simulink model "OA_Dynamic"  (R2020a)
settings: Solver=VariableStepAuto  StartTime=0.0  StopTime=30  RelTol=1e-3
values from neighbouring files (symbols this model uses):
  b = 0.4    [Takeoff.m]
  body_rate_0 = [0;0;0]    [Takeoff.m]
  Boundaries = [B1;B2;B3]    [Takeoff.m]
  Euler_0 = [0;0;0]    [Takeoff.m]
  g = [0;0;-9.8]    [Takeoff.m]
  I_Drone = [0.3933,0.3933,0.76]    [Takeoff.m]
  I_Tank = CalItank(m_tank,0.4,0.1,0.4,i)    [Takeoff.m]
  J = 0.00062    [Takeoff.m]
  K = 0.074    [Takeoff.m]
  k_T = MaxMotorThrsut/(MaxRPM^2)    (= 6.99167657551e-06)    [Takeoff.m]
  k_Thrsut2Torque = 0.021    [Takeoff.m]
  l = 0.5    [Takeoff.m]
  L = sqrt((x2-x1)^2 + (y2-y1)^2)    [Takeoff.m]
  m = m_drone + m_tank*percent    (= 36)    [Takeoff.m]    (also in animation.m = T_V1toI*T_V2toV1*T_BtoV2)
  m_drone = 20    [Takeoff.m]
  m_tank = 16    [Takeoff.m]
  MaxThrust = 4*MaxMotorThrsut    (= 529.2)    [Takeoff.m]
  MaxTilt = 30*pi/180    (= 0.523598775598)    [Takeoff.m]
  MaxTorque_XY = (T2-T1)*(l/sqrt(2))    [Takeoff.m]
  MaxVolt = 48    [Takeoff.m]
  MaxYawRate = 100*pi/180    (= 1.74532925199)    [Takeoff.m]
  MaxZVel = 2    [Takeoff.m]
  percent = 1    [Takeoff.m]
  Px1 = 0.2    [Takeoff.m]
  Pz1 = 1    [Takeoff.m]
  Pz2 = 100    [Takeoff.m]
  R = 0.0062    [Takeoff.m]
  RecObstacle = [[5,4,3] ... (first row only)    [Takeoff.m]
  SafeZone = 1.0    (= 1)    [Takeoff.m]
  Target = WayPts(3,:)    [Takeoff.m]
  ts = 0.01    [Takeoff.m]
  WayPts = [[XYZ_0(1) XYZ_0(2) XYZ_0(3)] ... (first row only)    [Takeoff.m]
  XYZ_0 = [0;0;0]    [Takeoff.m]
undefined symbols (not defined in the file or in its folder): b_tank, d_drone, d_tank, DiscIntNeverNeededParam, FlyVel, h_tank, PD1, PD2, PI1, PI2, PP1, PP2, SafeFactor, Sensor0Dir, TestVel
libraries: simulink x27, vrlib x4
(part 1 of 3)
settings Model: NumberOfSteps=10  Creator=blaze8871  LastModifiedBy=blaze8871
settings DataIOCC: SaveTime=off

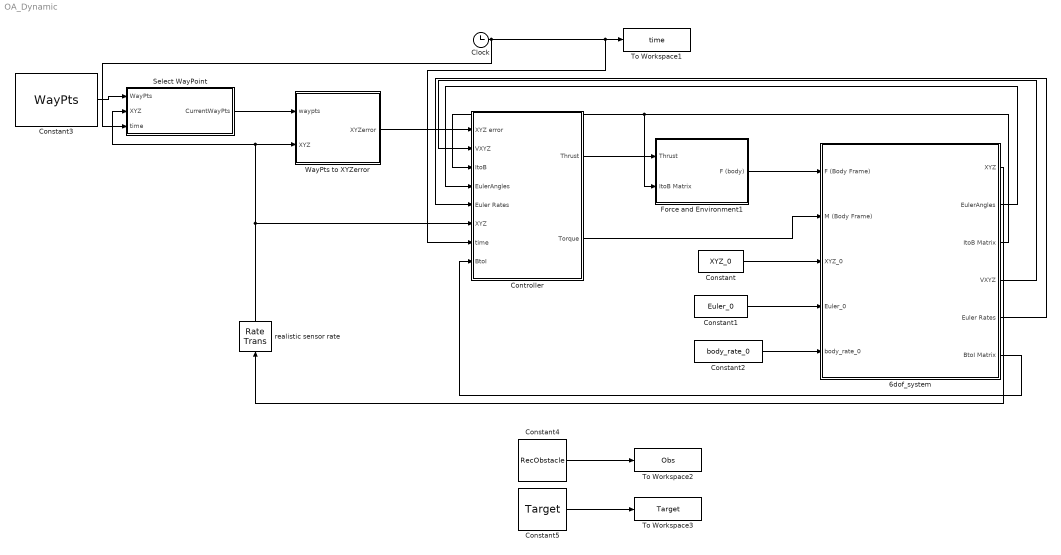
== system OA_Dynamic ==
  6dof_system : Subsystem
  Clock : Clock
  Constant : Constant  Value=XYZ_0  SampleTime=-1
  Constant1 : Constant  Value=Euler_0  SampleTime=-1
  Constant2 : Constant  Value=body_rate_0  SampleTime=-1
  Constant3 : Constant  Value=WayPts
  Constant4 : Constant  Value=RecObstacle
  Constant5 : Constant  Value=Target
  Controller : Subsystem
  Force and Environment1 : Subsystem
  Select WayPoint : Subsystem
  To Workspace1 : ToWorkspace  VariableName=time  SampleTime=ts
  To Workspace2 : ToWorkspace  VariableName=Obs  SampleTime=1000
  To Workspace3 : ToWorkspace  VariableName=Target  SampleTime=1000
  WayPts to XYZerror : MATLAB Function  TreatAsAtomicUnit=on
  realistic sensor rate : RateTransition  OutPortSampleTime=ts
  wires:
  Constant/1 -> 6dof_system/3(XYZ_0)
  Constant1/1 -> 6dof_system/4(Euler_0)
  Constant2/1 -> 6dof_system/5(body_rate_0)
  6dof_system/1(XYZ) -> realistic sensor rate/1
  6dof_system/2(EulerAngles) -> Controller/4(EulerAngles)
  WayPts to XYZerror/1(XYZerror) -> Controller/1(XYZ error)
  6dof_system/4(VXYZ) -> Controller/2(VXYZ)
  6dof_system/5(Euler Rates) -> Controller/5(Euler Rates)
  6dof_system/3(ItoB Matrix) -> Force and Environment1/2(ItoB Matrix), Controller/3(ItoB)
  Clock/1 -> Select WayPoint/3(time), Controller/7(time), To Workspace1/1
  Constant3/1 -> Select WayPoint/1(WayPts)
  realistic sensor rate/1 -> Select WayPoint/2(XYZ), WayPts to XYZerror/2(XYZ), Controller/6(XYZ)
  Select WayPoint/1(CurrentWayPts) -> WayPts to XYZerror/1(waypts)
  6dof_system/6(BtoI Matrix) -> Controller/8(BtoI)
  Controller/1(Thrust) -> Force and Environment1/1(Thrust)
  Force and Environment1/1(F (body)) -> 6dof_system/1(F (Body Frame))
  Controller/2(Torque) -> 6dof_system/2(M (Body Frame))
  Constant4/1 -> To Workspace2/1
  Constant5/1 -> To Workspace3/1

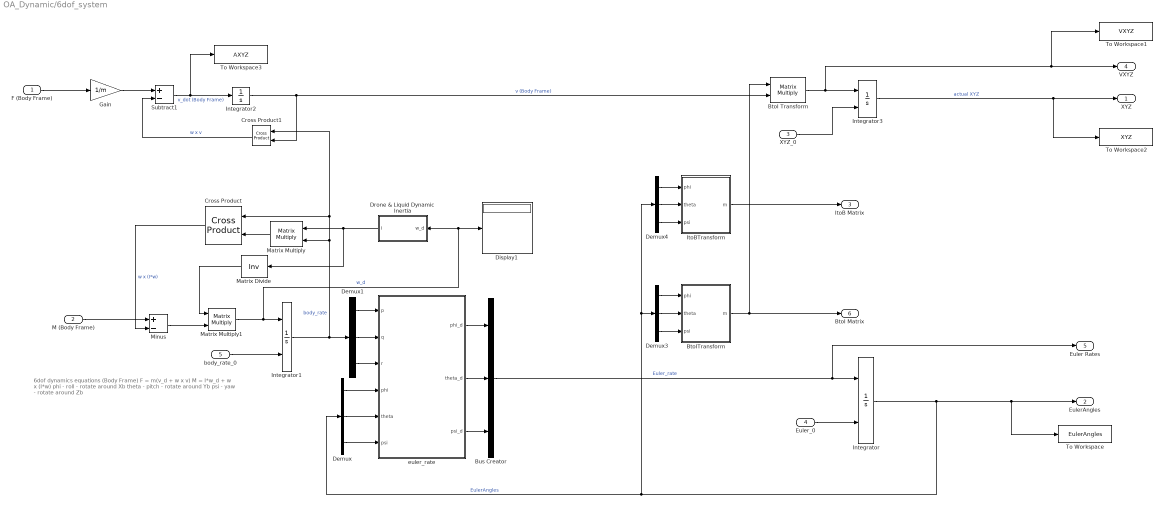
== system OA_Dynamic/6dof_system ==
  note: 6dof dynamics equations
      | (Body Frame)
      |
      | F = m(v_d + w x v)
      | M = I*w_d + w x (I*w)
      |
      | phi - roll - rotate around Xb
      | theta - pitch - rotate around Yb
      | psi - yaw - rotate around Zb
  F (Body Frame) : Inport
  M (Body Frame) : Inport  Port=2
  XYZ_0 : Inport  Port=3
  Euler_0 : Inport  Port=4
  body_rate_0 : Inport  Port=5
  BtoI Transform : Product  Multiplication=Matrix(*)
  BtoITransform : MATLAB Function  TreatAsAtomicUnit=on
  Bus Creator : BusCreator  Inputs=3
  Cross Product : vrlib/Utilities/Cross Product
  Cross Product1 : vrlib/Utilities/Cross Product
  Demux{,1,3..4} (4 alike) : Demux  Outputs=3
  Display1 : Display
  Drone & Liquid Dynamic Inertia : Subsystem
  Gain : Gain  Gain=1/m
  Integrator : Integrator  InitialConditionSource=external  ContinuousStateAttributes='EulerAngle'
  Integrator1 : Integrator  InitialConditionSource=external  ContinuousStateAttributes='EulerAngle'
  Integrator2 : Integrator
  Integrator3 : Integrator  InitialConditionSource=external
  ItoBTransform : MATLAB Function  TreatAsAtomicUnit=on
  Matrix Divide : Product  Inputs=/  Multiplication=Matrix(*)
  Matrix Multiply : Product  Multiplication=Matrix(*)
  Matrix Multiply1 : Product  Multiplication=Matrix(*)
  Minus : Sum  Inputs=+-
  Subtract1 : Sum  Inputs=+-
  To Workspace : ToWorkspace  VariableName=EulerAngles  SampleTime=ts
  To Workspace1 : ToWorkspace  VariableName=VXYZ  SampleTime=ts
  To Workspace2 : ToWorkspace  VariableName=XYZ  SampleTime=ts
  To Workspace3 : ToWorkspace  VariableName=AXYZ  SampleTime=ts
  euler_rate : MATLAB Function  TreatAsAtomicUnit=on
  XYZ : Outport
  EulerAngles : Outport  Port=2
  ItoB Matrix : Outport  Port=3
  VXYZ : Outport  Port=4
  Euler Rates : Outport  Port=5
  BtoI Matrix : Outport  Port=6
  wires:
  F (Body Frame)/1 -> Gain/1
  Demux4/2 -> ItoBTransform/2(theta)
  euler_rate/1(phi_d) -> Bus Creator/1
  BtoITransform/1(m) -> BtoI Matrix/1, BtoI Transform/1
  Bus Creator/1 -> Euler Rates/1, Integrator/1  "Euler_rate"
  Matrix Multiply/1 -> Cross Product/2
  Demux3/2 -> BtoITransform/2(theta)
  Demux/2 -> euler_rate/5(theta)
  Demux4/1 -> ItoBTransform/1(phi)
  Subtract1/1 -> To Workspace3/1, Integrator2/1  "v_dot (Body Frame)"
  Cross Product1/1 -> Subtract1/2  "w x v"
  Demux1/1 -> euler_rate/1(p)
  Demux/3 -> euler_rate/6(psi)
  euler_rate/2(theta_d) -> Bus Creator/2
  Euler_0/1 -> Integrator/2
  Integrator3/1 -> To Workspace2/1, XYZ/1  "actual XYZ"
  Cross Product/1 -> Minus/2  "w x (I*w)"
  M (Body Frame)/1 -> Minus/1
  body_rate_0/1 -> Integrator1/2
  Demux3/3 -> BtoITransform/3(psi)
  euler_rate/3(psi_d) -> Bus Creator/3
  Demux4/3 -> ItoBTransform/3(psi)
  Gain/1 -> Subtract1/1
  Demux3/1 -> BtoITransform/1(phi)
  Demux1/3 -> euler_rate/3(r)
  XYZ_0/1 -> Integrator3/2
  Demux/1 -> euler_rate/4(phi)
  Integrator2/1 -> Cross Product1/2, BtoI Transform/2  "v (Body Frame)"
  Integrator1/1 -> Cross Product1/1, Cross Product/1, Matrix Multiply/2, Demux1/1  "body_rate"
  Demux1/2 -> euler_rate/2(q)
  ItoBTransform/1(m) -> ItoB Matrix/1
  BtoI Transform/1 -> To Workspace1/1, VXYZ/1, Integrator3/1
  Minus/1 -> Matrix Multiply1/2
  Matrix Multiply1/1 -> Integrator1/1, Display1/1, Drone & Liquid Dynamic Inertia/1(w_d)  "w_d"
  Integrator/1 -> To Workspace/1, EulerAngles/1, Demux4/1, Demux3/1, Demux/1  "EulerAngles"
  Drone & Liquid Dynamic Inertia/1(I) -> Matrix Divide/1, Matrix Multiply/1
  Matrix Divide/1 -> Matrix Multiply1/1

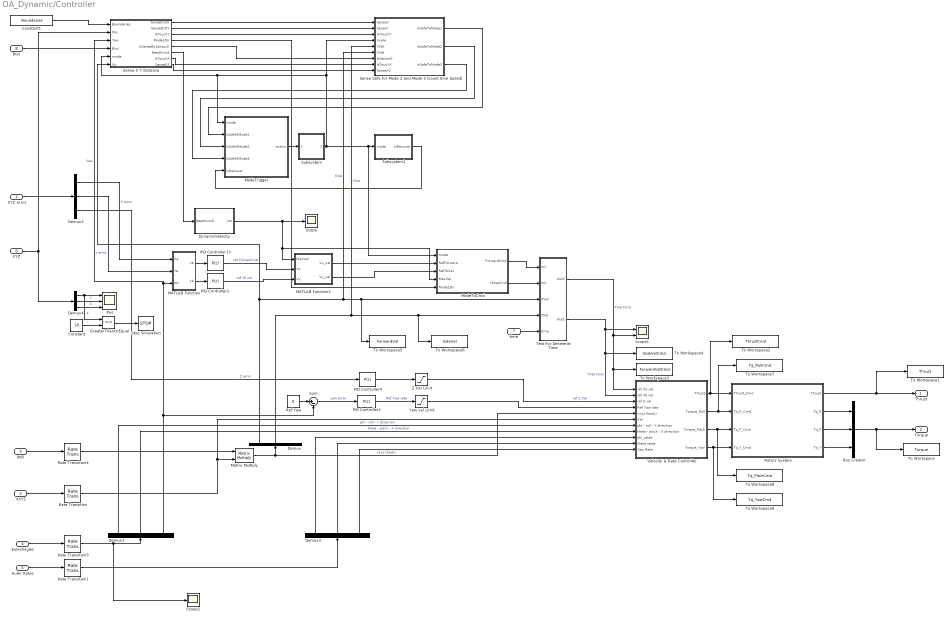
== system OA_Dynamic/Controller ==
  XYZ error : Inport
  VXYZ : Inport  Port=2
  ItoB : Inport  Port=3
  EulerAngles : Inport  Port=4
  Euler Rates : Inport  Port=5
  XYZ : Inport  Port=6
  time : Inport  Port=7
  BtoI : Inport  Port=8
  Bus Creator : BusCreator  Inputs=3
  Constant : Constant  Value=20
  Constant1 : Constant  Value=Boundaries
  Demux{,1..4} (5 alike) : Demux  Outputs=3
  DynamicVelocity : Subsystem
  GreaterThanOrEqual : RelationalOperator  OutDataTypeStr=boolean  RndMeth=Simplest
  MATLAB Function : MATLAB Function  TreatAsAtomicUnit=on
  MATLAB Function2 : MATLAB Function  TreatAsAtomicUnit=on
  Matrix Multiply : Product  Multiplication=Matrix(*)
  ModeToCmd : MATLAB Function  TreatAsAtomicUnit=on
  ModeTrigger : MATLAB Function  TreatAsAtomicUnit=on
  PID Controller1 : simulink/Continuous/PID Controller  Controller=P  Form=Parallel  TimeDomain=Discrete-time  UseExternalTs=off  SampleTime=ts  IntegratorMethod=Forward Euler  FilterMethod=Forward Euler  ControllerParametersSource=internal  P=1  I=1  D=0  UseFilter=on  N=100  TunerSelectOption=Transfer Function Based (PID Tuner App)  InitialConditionSource=internal  InitialConditionForIntegrator=0  InitialConditionForFilter=0  DifferentiatorICPrevScaledInput=0  ExternalReset=none  TrackingMode=off  Kt=1  LimitOutput=off  UpperSaturationLimit=inf  LowerSaturationLimit=-inf  LinearizeAsGain=on  AntiWindupMode=none  Kb=1  POutMin=[]  POutMax=[]  IOutMin=[]  IOutMax=[]  DOutMin=[]  DOutMax=[]  NOutMin=[]  NOutMax=[]  SumOutMin=[]  SumOutMax=[]  SaturationOutMin=[]  SaturationOutMax=[]  PParamMin=[]  PParamMax=[]  IParamMin=[]  IParamMax=[]  DParamMin=[]  DParamMax=[]  NParamMin=[]  NParamMax=[]  KbParamMin=[]  KbParamMax=[]  KtParamMin=[]  KtParamMax=[]  KbOutMin=[]  KbOutMax=[]  KtOutMin=[]  KtOutMax=[]  IntegratorOutMin=[]  IntegratorOutMax=[]  FilterOutMin=[]  FilterOutMax=[]  SumI1OutMin=[]  SumI1OutMax=[]  SumI2OutMin=[]  SumI2OutMax=[]  SumI3OutMin=[]  SumI3OutMax=[]  SumI4OutMin=[]  SumI4OutMax=[]  SumDOutMin=[]  SumDOutMax=[]  DifferentiatorOutMin=[]  DifferentiatorOutMax=[]  FilterDiffOutCoefMin=[]  FilterDiffOutCoefMax=[]  ReciprocalOutMin=[]  ReciprocalOutMax=[]  SumDenOutMin=[]  SumDenOutMax=[]  SumNumOutMin=[]  SumNumOutMax=[]  DivideOutMin=[]  DivideOutMax=[]  UdiffTsProdOutMin=[]  UdiffTsProdOutMax=[]  NTsProdOutMin=[]  NTsProdOutMax=[]  UintegralTsProdOutMin=[]  UintegralTsProdOutMax=[]  UngainTsProdOutMin=[]  UngainTsProdOutMax=[]  IntegratorContinuousStateAttributes=''  IntegratorStateMustResolveToSignalObject=off  IntegratorRTWStateStorageClass=Auto  FilterContinuousStateAttributes=''  FilterStateMustResolveToSignalObject=off  FilterRTWStateStorageClass=Auto  ParallelPVariant=InternalParameters  IdealPVariant=Disabled  IVariant=Disabled  DVariant=Disabled  IntegratorVariant=Disabled  SatVariant=Disabled  AWVariant=Disabled  PCopyVariant=Disabled  TRVariant=Disabled  FdbkBlocksVariant=Forward  IdealPFdbkVariant=Disabled  SatFdbkVariant=Disabled  DerivativeFilterVariant=Disabled  NVariant=Disabled  NCopyVariant=Disabled_SignalSpec  FilterICVariant=Disabled  IntegratorICVariant=Disabled  ExternalResetVariant=Disabled  TRSumVariant=Passthrough  SumFdbkVariant=Disabled  SumVariant=Passthrough_P  TsampFilterVariant=InternalTs  TsampNgainVariant=Passthrough  TsampIntegralVariant=Disabled_SignalSpec
  PID Controller13 : simulink/Continuous/PID Controller  Controller=P  Form=Parallel  TimeDomain=Discrete-time  UseExternalTs=off  SampleTime=ts  IntegratorMethod=Forward Euler  FilterMethod=Forward Euler  ControllerParametersSource=internal  P=0.6  I=1  D=0  UseFilter=on  N=100  TunerSelectOption=Transfer Function Based (PID Tuner App)  InitialConditionSource=internal  InitialConditionForIntegrator=0  InitialConditionForFilter=0  DifferentiatorICPrevScaledInput=0  ExternalReset=none  TrackingMode=off  Kt=1  LimitOutput=off  UpperSaturationLimit=inf  LowerSaturationLimit=-inf  LinearizeAsGain=on  AntiWindupMode=none  Kb=1  POutMin=[]  POutMax=[]  IOutMin=[]  IOutMax=[]  DOutMin=[]  DOutMax=[]  NOutMin=[]  NOutMax=[]  SumOutMin=[]  SumOutMax=[]  SaturationOutMin=[]  SaturationOutMax=[]  PParamMin=[]  PParamMax=[]  IParamMin=[]  IParamMax=[]  DParamMin=[]  DParamMax=[]  NParamMin=[]  NParamMax=[]  KbParamMin=[]  KbParamMax=[]  KtParamMin=[]  KtParamMax=[]  KbOutMin=[]  KbOutMax=[]  KtOutMin=[]  KtOutMax=[]  IntegratorOutMin=[]  IntegratorOutMax=[]  FilterOutMin=[]  FilterOutMax=[]  SumI1OutMin=[]  SumI1OutMax=[]  SumI2OutMin=[]  SumI2OutMax=[]  SumI3OutMin=[]  SumI3OutMax=[]  SumI4OutMin=[]  SumI4OutMax=[]  SumDOutMin=[]  SumDOutMax=[]  DifferentiatorOutMin=[]  DifferentiatorOutMax=[]  FilterDiffOutCoefMin=[]  FilterDiffOutCoefMax=[]  ReciprocalOutMin=[]  ReciprocalOutMax=[]  SumDenOutMin=[]  SumDenOutMax=[]  SumNumOutMin=[]  SumNumOutMax=[]  DivideOutMin=[]  DivideOutMax=[]  UdiffTsProdOutMin=[]  UdiffTsProdOutMax=[]  NTsProdOutMin=[]  NTsProdOutMax=[]  UintegralTsProdOutMin=[]  UintegralTsProdOutMax=[]  UngainTsProdOutMin=[]  UngainTsProdOutMax=[]  IntegratorContinuousStateAttributes=''  IntegratorStateMustResolveToSignalObject=off  IntegratorRTWStateStorageClass=Auto  FilterContinuousStateAttributes=''  FilterStateMustResolveToSignalObject=off  FilterRTWStateStorageClass=Auto  ParallelPVariant=InternalParameters  IdealPVariant=Disabled  IVariant=Disabled  DVariant=Disabled  IntegratorVariant=Disabled  SatVariant=Disabled  AWVariant=Disabled  PCopyVariant=Disabled  TRVariant=Disabled  FdbkBlocksVariant=Forward  IdealPFdbkVariant=Disabled  SatFdbkVariant=Disabled  DerivativeFilterVariant=Disabled  NVariant=Disabled  NCopyVariant=Disabled_SignalSpec  FilterICVariant=Disabled  IntegratorICVariant=Disabled  ExternalResetVariant=Disabled  TRSumVariant=Passthrough  SumFdbkVariant=Disabled  SumVariant=Passthrough_P  TsampFilterVariant=InternalTs  TsampNgainVariant=Passthrough  TsampIntegralVariant=Disabled_SignalSpec
  PID Controller2 : simulink/Continuous/PID Controller  Controller=P  Form=Parallel  TimeDomain=Discrete-time  UseExternalTs=off  SampleTime=ts  IntegratorMethod=Forward Euler  FilterMethod=Forward Euler  ControllerParametersSource=internal  P=0.6  I=1  D=0  UseFilter=on  N=100  TunerSelectOption=Transfer Function Based (PID Tuner App)  InitialConditionSource=internal  InitialConditionForIntegrator=0  InitialConditionForFilter=0  DifferentiatorICPrevScaledInput=0  ExternalReset=none  TrackingMode=off  Kt=1  LimitOutput=off  UpperSaturationLimit=inf  LowerSaturationLimit=-inf  LinearizeAsGain=on  AntiWindupMode=none  Kb=1  POutMin=[]  POutMax=[]  IOutMin=[]  IOutMax=[]  DOutMin=[]  DOutMax=[]  NOutMin=[]  NOutMax=[]  SumOutMin=[]  SumOutMax=[]  SaturationOutMin=[]  SaturationOutMax=[]  PParamMin=[]  PParamMax=[]  IParamMin=[]  IParamMax=[]  DParamMin=[]  DParamMax=[]  NParamMin=[]  NParamMax=[]  KbParamMin=[]  KbParamMax=[]  KtParamMin=[]  KtParamMax=[]  KbOutMin=[]  KbOutMax=[]  KtOutMin=[]  KtOutMax=[]  IntegratorOutMin=[]  IntegratorOutMax=[]  FilterOutMin=[]  FilterOutMax=[]  SumI1OutMin=[]  SumI1OutMax=[]  SumI2OutMin=[]  SumI2OutMax=[]  SumI3OutMin=[]  SumI3OutMax=[]  SumI4OutMin=[]  SumI4OutMax=[]  SumDOutMin=[]  SumDOutMax=[]  DifferentiatorOutMin=[]  DifferentiatorOutMax=[]  FilterDiffOutCoefMin=[]  FilterDiffOutCoefMax=[]  ReciprocalOutMin=[]  ReciprocalOutMax=[]  SumDenOutMin=[]  SumDenOutMax=[]  SumNumOutMin=[]  SumNumOutMax=[]  DivideOutMin=[]  DivideOutMax=[]  UdiffTsProdOutMin=[]  UdiffTsProdOutMax=[]  NTsProdOutMin=[]  NTsProdOutMax=[]  UintegralTsProdOutMin=[]  UintegralTsProdOutMax=[]  UngainTsProdOutMin=[]  UngainTsProdOutMax=[]  IntegratorContinuousStateAttributes=''  IntegratorStateMustResolveToSignalObject=off  IntegratorRTWStateStorageClass=Auto  FilterContinuousStateAttributes=''  FilterStateMustResolveToSignalObject=off  FilterRTWStateStorageClass=Auto  ParallelPVariant=InternalParameters  IdealPVariant=Disabled  IVariant=Disabled  DVariant=Disabled  IntegratorVariant=Disabled  SatVariant=Disabled  AWVariant=Disabled  PCopyVariant=Disabled  TRVariant=Disabled  FdbkBlocksVariant=Forward  IdealPFdbkVariant=Disabled  SatFdbkVariant=Disabled  DerivativeFilterVariant=Disabled  NVariant=Disabled  NCopyVariant=Disabled_SignalSpec  FilterICVariant=Disabled  IntegratorICVariant=Disabled  ExternalResetVariant=Disabled  TRSumVariant=Passthrough  SumFdbkVariant=Disabled  SumVariant=Passthrough_P  TsampFilterVariant=InternalTs  TsampNgainVariant=Passthrough  TsampIntegralVariant=Disabled_SignalSpec
  PID Controller4 : simulink/Continuous/PID Controller  Controller=P  Form=Parallel  TimeDomain=Discrete-time  UseExternalTs=off  SampleTime=ts  IntegratorMethod=Forward Euler  FilterMethod=Forward Euler  ControllerParametersSource=internal  P=Pz1  I=1  D=0  UseFilter=on  N=100  TunerSelectOption=Transfer Function Based (PID Tuner App)  InitialConditionSource=internal  InitialConditionForIntegrator=0  InitialConditionForFilter=0  DifferentiatorICPrevScaledInput=0  ExternalReset=none  TrackingMode=off  Kt=1  LimitOutput=off  UpperSaturationLimit=inf  LowerSaturationLimit=-inf  LinearizeAsGain=on  AntiWindupMode=none  Kb=1  POutMin=[]  POutMax=[]  IOutMin=[]  IOutMax=[]  DOutMin=[]  DOutMax=[]  NOutMin=[]  NOutMax=[]  SumOutMin=[]  SumOutMax=[]  SaturationOutMin=[]  SaturationOutMax=[]  PParamMin=[]  PParamMax=[]  IParamMin=[]  IParamMax=[]  DParamMin=[]  DParamMax=[]  NParamMin=[]  NParamMax=[]  KbParamMin=[]  KbParamMax=[]  KtParamMin=[]  KtParamMax=[]  KbOutMin=[]  KbOutMax=[]  KtOutMin=[]  KtOutMax=[]  IntegratorOutMin=[]  IntegratorOutMax=[]  FilterOutMin=[]  FilterOutMax=[]  SumI1OutMin=[]  SumI1OutMax=[]  SumI2OutMin=[]  SumI2OutMax=[]  SumI3OutMin=[]  SumI3OutMax=[]  SumI4OutMin=[]  SumI4OutMax=[]  SumDOutMin=[]  SumDOutMax=[]  DifferentiatorOutMin=[]  DifferentiatorOutMax=[]  FilterDiffOutCoefMin=[]  FilterDiffOutCoefMax=[]  ReciprocalOutMin=[]  ReciprocalOutMax=[]  SumDenOutMin=[]  SumDenOutMax=[]  SumNumOutMin=[]  SumNumOutMax=[]  DivideOutMin=[]  DivideOutMax=[]  UdiffTsProdOutMin=[]  UdiffTsProdOutMax=[]  NTsProdOutMin=[]  NTsProdOutMax=[]  UintegralTsProdOutMin=[]  UintegralTsProdOutMax=[]  UngainTsProdOutMin=[]  UngainTsProdOutMax=[]  IntegratorContinuousStateAttributes=''  IntegratorStateMustResolveToSignalObject=off  IntegratorRTWStateStorageClass=Auto  FilterContinuousStateAttributes=''  FilterStateMustResolveToSignalObject=off  FilterRTWStateStorageClass=Auto  ParallelPVariant=InternalParameters  IdealPVariant=Disabled  IVariant=Disabled  DVariant=Disabled  IntegratorVariant=Disabled  SatVariant=Disabled  AWVariant=Disabled  PCopyVariant=Disabled  TRVariant=Disabled  FdbkBlocksVariant=Forward  IdealPFdbkVariant=Disabled  SatFdbkVariant=Disabled  DerivativeFilterVariant=Disabled  NVariant=Disabled  NCopyVariant=Disabled_SignalSpec  FilterICVariant=Disabled  IntegratorICVariant=Disabled  ExternalResetVariant=Disabled  TRSumVariant=Passthrough  SumFdbkVariant=Disabled  SumVariant=Passthrough_P  TsampFilterVariant=InternalTs  TsampNgainVariant=Passthrough  TsampIntegralVariant=Disabled_SignalSpec
  Pos : Scope  NumInputPorts=3
  Rate Transition{,1,3..4} (4 alike) : RateTransition  OutPortSampleTime=ts
  Ref Yaw : Constant  Value=0
  Rotors System : Subsystem
  Scope : Scope
  Scope1 : Scope  NumInputPorts=2
  Scope2 : Scope
  Sense Safe for Mode 2 and Mode 3 (count time based) : Subsystem
  Sense X Y Distance : Subsystem
  Stop Simulation : Stop
  Subsystem : Subsystem
  Subsystem1 : Subsystem
  Sum : Sum  Inputs=|+-
  Test For Decelerat Time : Subsystem
  To Workspace : ToWorkspace  VariableName=Torque  SampleTime=ts
  To Workspace1 : ToWorkspace  VariableName=Thrust  SampleTime=ts
  To Workspace2 : ToWorkspace  VariableName=ThrustCmd  SampleTime=ts
  To Workspace3 : ToWorkspace  VariableName=ForwardVelCmd  SampleTime=ts
  To Workspace4 : ToWorkspace  VariableName=SideVelCmd  SampleTime=ts
  To Workspace5 : ToWorkspace  VariableName=ForwardVel  SampleTime=ts
  To Workspace6 : ToWorkspace  VariableName=SideVel  SampleTime=ts
  To Workspace7 : ToWorkspace  VariableName=Tq_RollCmd  SampleTime=ts
  To Workspace8 : ToWorkspace  VariableName=Tq_PitchCmd  SampleTime=ts
  To Workspace9 : ToWorkspace  VariableName=Tq_YawCmd  SampleTime=ts
  Velocity & Rate Controller : Subsystem
  Yaw vel Limit : Saturate  UpperLimit=MaxYawRate  LowerLimit=-MaxYawRate
  Z Vel Limit : Saturate  UpperLimit=MaxZVel  LowerLimit=-MaxZVel
  Thrust : Outport
  Torque : Outport  Port=2
  wires:
  Bus Creator/1 -> To Workspace/1, Torque/1
  VXYZ/1 -> Rate Transition/1
  Demux2/3 -> PID Controller4/1  "Z error"
  EulerAngles/1 -> Rate Transition3/1
  Demux1/3 -> MATLAB Function/3(psi), Sense X Y Distance/3(Yaw), Sum/2  "Yaw"
  Sum/1 -> PID Controller1/1  "yaw error"
  ItoB/1 -> Rate Transition4/1
  XYZ error/1 -> Demux2/1
  Rate Transition3/1 -> Scope2/1, Demux1/1
  Rate Transition4/1 -> Matrix Multiply/1
  Euler Rates/1 -> Rate Transition1/1
  Rate Transition1/1 -> Demux3/1
  Demux2/1 -> MATLAB Function/1(Xe)  "X error"
  Demux2/2 -> MATLAB Function/2(Ye)  "y error"
  Rate Transition/1 -> Velocity & Rate Controller/6(Vel), Matrix Multiply/2
  MATLAB Function/1(xb) -> PID Controller13/1
  PID Controller13/1 -> MATLAB Function2/2(Vx)  "ref Forward vel"
  Matrix Multiply/1 -> Velocity & Rate Controller/5(vxyz (body)), Demux/1  "vxyz (body)"
  PID Controller4/1 -> Z Vel Limit/1
  PID Controller1/1 -> Yaw vel Limit/1  "Ref Yaw rate"
  Demux1/1 -> Velocity & Rate Controller/7(phi - roll - Y direction)  "phi - roll - Y direction"
  Demux1/2 -> Velocity & Rate Controller/8(theta - pitch - X direction)  "theta - pitch - X direction"
  Demux3/1 -> Velocity & Rate Controller/9(phi_rates)
  Demux3/2 -> Velocity & Rate Controller/10(theta rates)
  Demux3/3 -> Velocity & Rate Controller/11(Yaw Rate)
  MATLAB Function2/1(Vx_cal) -> ModeToCmd/2(RefForward)
  Yaw vel Limit/1 -> Velocity & Rate Controller/4(Ref Yaw rate)
  Ref Yaw/1 -> Sum/1
  MATLAB Function/2(yb) -> PID Controller2/1
  PID Controller2/1 -> MATLAB Function2/3(Vy)  "ref Yb vel"
  MATLAB Function2/2(Vy_cal) -> ModeToCmd/3(RefYbVel)
  XYZ/1 -> Sense X Y Distance/2(Pos), Demux4/1
  Demux4/1 -> GreaterThanOrEqual/1, Pos/1  "X"
  Demux4/2 -> Pos/2  "Y"
  Demux4/3 -> Pos/3  "Z"
  Demux/2 -> Sense Safe for Mode 2 and Mode 3 (count time based)/5(YVel), To Workspace6/1, Test For Decelerat Time/4(YVel)  "YVel"
  Demux/1 -> Sense X Y Distance/6(Vx), Sense Safe for Mode 2 and Mode 3 (count time based)/6(XVel), To Workspace5/1, Test For Decelerat Time/3(XVel)  "XVel"
  Sense X Y Distance/1(SenseDistX) -> Sense Safe for Mode 2 and Mode 3 (count time based)/1(SenseX)
  Constant1/1 -> Sense X Y Distance/1(Boundaries)
  Sense X Y Distance/2(SenseDistY) -> Sense Safe for Mode 2 and Mode 3 (count time based)/2(SenseY)
  Velocity & Rate Controller/1(Thrust) -> Rotors System/1(Thrust_Cmd), To Workspace2/1
  Velocity & Rate Controller/2(Torque_Roll) -> To Workspace7/1, Rotors System/2(Tq_R_Cmd)
  Velocity & Rate Controller/3(Torque_Pitch) -> To Workspace8/1, Rotors System/3(Tq_P_Cmd)
  Velocity & Rate Controller/4(Torque_Yaw) -> To Workspace9/1, Rotors System/4(Tq_Y_Cmd)
  Rotors System/1(Thrust) -> Thrust/1, To Workspace1/1
  Rotors System/2(Tq_R) -> Bus Creator/1
  Rotors System/3(Tq_P) -> Bus Creator/2
  Rotors System/4(Tq_Y) -> Bus Creator/3
  Subsystem/1(mode) -> Subsystem1/1(mode), ModeToCmd/1(mode), ModeTrigger/1(mode), Sense X Y Distance/5(mode), Sense Safe for Mode 2 and Mode 3 (count time based)/4(mode)
  ModeTrigger/1(action) -> Subsystem/1(action)
  Subsystem1/1(IsRecover) -> ModeTrigger/5(IsRecover)
  Z Vel Limit/1 -> Velocity & Rate Controller/3(ref Z vel)  "ref Z Vel"
  Sense Safe for Mode 2 and Mode 3 (count time based)/2(IsSafeToMode2) -> ModeTrigger/3(IsSafe2Mode2)
  Sense X Y Distance/3(IsTouchY) -> Sense Safe for Mode 2 and Mode 3 (count time based)/3(IsTouchY)
  Sense Safe for Mode 2 and Mode 3 (count time based)/3(IsSafeToMode3) -> ModeTrigger/4(IsSafe2Mode3)
  Test For Decelerat Time/2(Out1) -> Scope1/1, To Workspace4/1, Velocity & Rate Controller/2(ref Yb vel)  "YVel Cmd"
  Test For Decelerat Time/1(Out2) -> Scope1/2, To Workspace3/1, Velocity & Rate Controller/1(ref Xb vel)  "XVel Cmd"
  ModeToCmd/1(ForwardCmd) -> Test For Decelerat Time/1(In1)
  ModeToCmd/2(YbVelCmd) -> Test For Decelerat Time/2(In2)
  time/1 -> Test For Decelerat Time/5(time)
  Sense Safe for Mode 2 and Mode 3 (count time based)/1(IsSafeToMode1) -> ModeTrigger/2(IsSafe2Mode1)
  BtoI/1 -> Sense X Y Distance/4(BtoI)
  Sense X Y Distance/4(Mode1Dir) -> ModeToCmd/5(Mode1Dir)
  Sense X Y Distance/5(IsSenseBySensor0) -> Sense Safe for Mode 2 and Mode 3 (count time based)/7(IsSensor0)
  DynamicVelocity/1(Vel) -> Scope/1, ModeToCmd/4(MaxVel), MATLAB Function2/1(MaxVel)
  Sense X Y Distance/6(NeedAvoid) -> DynamicVelocity/1(NeedAvoid)
  Sense X Y Distance/7(IsTouchX) -> Sense Safe for Mode 2 and Mode 3 (count time based)/8(IsTouchX)
  Sense X Y Distance/8(SenseX2) -> Sense Safe for Mode 2 and Mode 3 (count time based)/9(SenseX2)
  GreaterThanOrEqual/1 -> Stop Simulation/1
  Constant/1 -> GreaterThanOrEqual/2

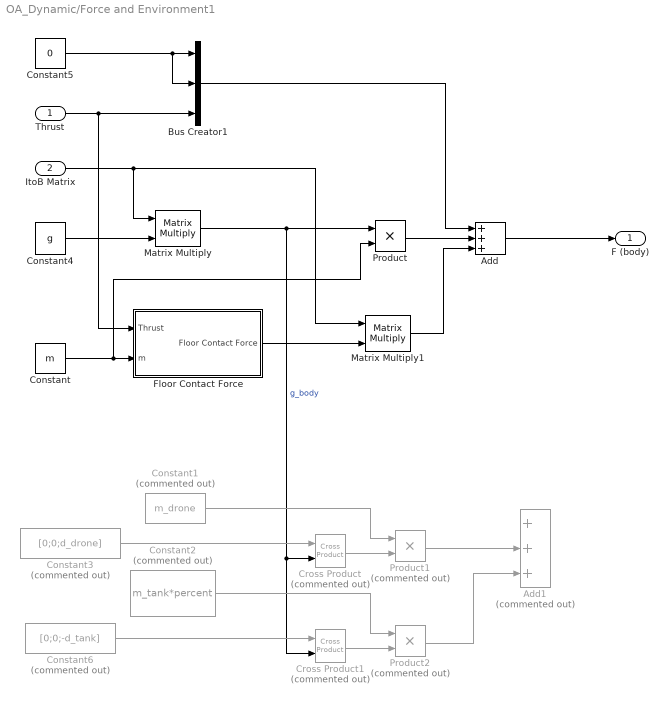
== system OA_Dynamic/Force and Environment1 ==
  Thrust : Inport
  ItoB Matrix : Inport  Port=2
  Add : Sum  Inputs=+++
  Add1 : Sum  Commented=on  Inputs=+++
  Bus Creator1 : BusCreator  Inputs=3
  Constant : Constant  Value=m  SampleTime=ts
  Constant1 : Constant  Commented=on  Value=m_drone  SampleTime=ts
  Constant2 : Constant  Commented=on  Value=m_tank*percent  SampleTime=ts
  Constant3 : Constant  Commented=on  Value=[0;0;d_drone]  SampleTime=ts
  Constant4 : Constant  Value=g  SampleTime=-1
  Constant5 : Constant  Value=0  SampleTime=-1
  Constant6 : Constant  Commented=on  Value=[0;0;-d_tank]  SampleTime=ts
  Cross Product : vrlib/Utilities/Cross Product  Commented=on
  Cross Product1 : vrlib/Utilities/Cross Product  Commented=on
  Floor Contact Force : Subsystem
  Matrix Multiply : Product  Multiplication=Matrix(*)
  Matrix Multiply1 : Product  Multiplication=Matrix(*)
  Product : Product
  Product1 : Product  Commented=on
  Product2 : Product  Commented=on
  F (body) : Outport
  wires:
  Thrust/1 -> Floor Contact Force/1(Thrust), Bus Creator1/3
  ItoB Matrix/1 -> Matrix Multiply/1, Matrix Multiply1/1
  Constant5/1 -> Bus Creator1/2, Bus Creator1/1
  Add/1 -> F (body)/1
  Constant/1 -> Product/2, Floor Contact Force/2(m)
  Bus Creator1/1 -> Add/1
  Floor Contact Force/1(Floor Contact Force) -> Matrix Multiply1/2
  Matrix Multiply1/1 -> Add/3
  Constant4/1 -> Matrix Multiply/2
  Matrix Multiply/1 -> Cross Product/2, Cross Product1/2, Product/1  "g_body"
  Product/1 -> Add/2
  Constant3/1 -> Cross Product/1
  Cross Product/1 -> Product1/2
  Constant1/1 -> Product1/1
  Cross Product1/1 -> Product2/2
  Constant6/1 -> Cross Product1/1
  Constant2/1 -> Product2/1
  Product1/1 -> Add1/2
  Product2/1 -> Add1/3

== system OA_Dynamic/Select WayPoint ==
  WayPts : Inport
  XYZ : Inport  Port=2
  time : Inport  Port=3
  Discrete-Time Integrator : DiscreteIntegrator  SampleTime=ts  ICPrevOutput=DiscIntNeverNeededParam  ICPrevScaledInput=DiscIntNeverNeededParam
  Gain : Gain  Gain=100
  MATLAB Function : MATLAB Function  TreatAsAtomicUnit=on
  MATLAB Function1 : MATLAB Function  TreatAsAtomicUnit=on
  Scope : Scope
  CurrentWayPts : Outport
  wires:
  WayPts/1 -> MATLAB Function/1(WayPts)
  MATLAB Function/1(CurrentWayPts) -> CurrentWayPts/1, MATLAB Function1/1(CurrentWayPts)
  Gain/1 -> MATLAB Function1/3(Index), MATLAB Function/2(WayPtsIndex), Scope/1
  XYZ/1 -> MATLAB Function1/2(XYZ)
  MATLAB Function1/1(TouchWayPts) -> Discrete-Time Integrator/1
  Discrete-Time Integrator/1 -> Gain/1
  time/1 -> MATLAB Function1/4(time)

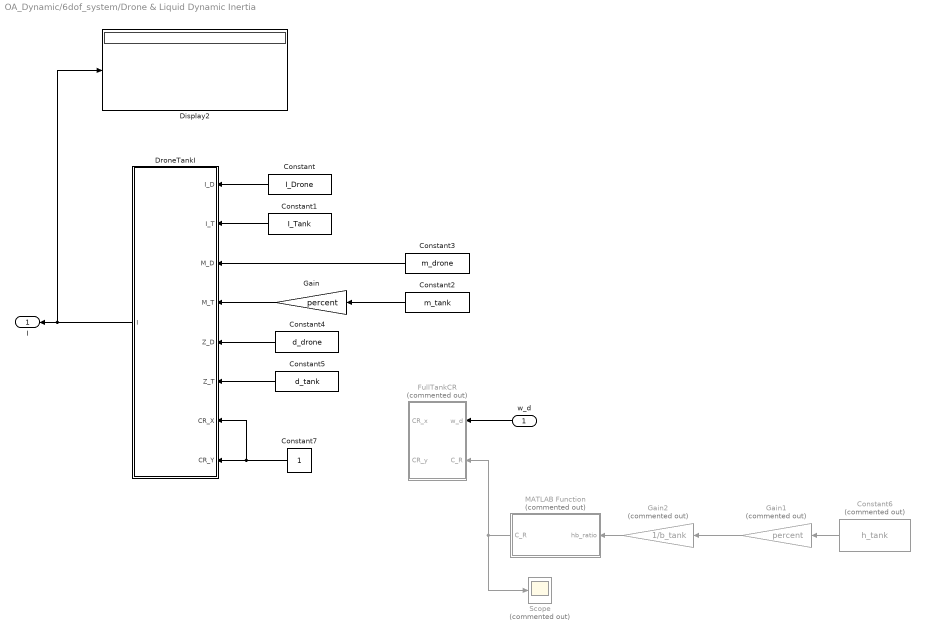
== system OA_Dynamic/6dof_system/Drone & Liquid Dynamic Inertia ==
  w_d : Inport
  Constant : Constant  Value=I_Drone
  Constant1 : Constant  Value=I_Tank
  Constant2 : Constant  Value=m_tank
  Constant3 : Constant  Value=m_drone
  Constant4 : Constant  Value=d_drone
  Constant5 : Constant  Value=d_tank
  Constant6 : Constant  Commented=on  Value=h_tank
  Constant7 : Constant
  Display2 : Display
  DroneTankI : MATLAB Function  TreatAsAtomicUnit=on
  FullTankCR : MATLAB Function  Commented=on  TreatAsAtomicUnit=on
  Gain : Gain  Gain=percent
  Gain1 : Gain  Commented=on  Gain=percent
  Gain2 : Gain  Commented=on  Gain=1/b_tank
  MATLAB Function : MATLAB Function  Commented=on  TreatAsAtomicUnit=on
  Scope : Scope  Commented=on
  I : Outport
  wires:
  Constant/1 -> DroneTankI/1(I_D)
  w_d/1 -> FullTankCR/1(w_d)
  DroneTankI/1(I) -> Display2/1, I/1
  Constant1/1 -> DroneTankI/2(I_T)
  Constant3/1 -> DroneTankI/3(M_D)
  Gain/1 -> DroneTankI/4(M_T)
  Constant2/1 -> Gain/1
  Constant4/1 -> DroneTankI/5(Z_D)
  Constant5/1 -> DroneTankI/6(Z_T)
  Constant6/1 -> Gain1/1
  Gain1/1 -> Gain2/1
  Gain2/1 -> MATLAB Function/1(hb_ratio)
  MATLAB Function/1(C_R) -> Scope/1, FullTankCR/2(C_R)
  Constant7/1 -> DroneTankI/8(CR_Y), DroneTankI/7(CR_X)

== system OA_Dynamic/Controller/DynamicVelocity ==
  NeedAvoid : Inport
  Constant : Constant  Value=percent
  Constant2 : Constant  Value=FlyVel
  MATLAB Function1 : MATLAB Function  TreatAsAtomicUnit=on
  MATLAB Function3 : MATLAB Function  TreatAsAtomicUnit=on
  To Workspace2 : ToWorkspace  VariableName=P_LQ  SampleTime=1000
  Vel : Outport
  wires:
  MATLAB Function3/1(Vel) -> Vel/1
  NeedAvoid/1 -> MATLAB Function3/1(NeedAvoid)
  Constant2/1 -> MATLAB Function3/2(FlyVel)
  MATLAB Function1/1(MaxVel) -> MATLAB Function3/3(MaxVel)
  Constant/1 -> To Workspace2/1, MATLAB Function1/1(WaterLevel)

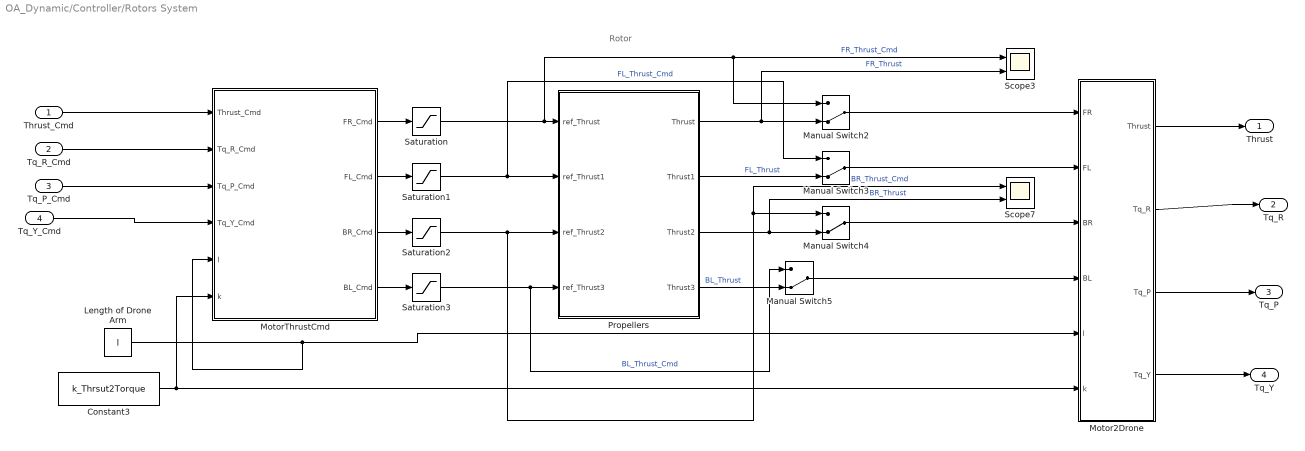
== system OA_Dynamic/Controller/Rotors System ==
  note: Rotor
  Thrust_Cmd : Inport
  Tq_R_Cmd : Inport  Port=2
  Tq_P_Cmd : Inport  Port=3
  Tq_Y_Cmd : Inport  Port=4
  Constant3 : Constant  Value=k_Thrsut2Torque
  Length of Drone Arm : Constant  Value=l
  Manual Switch{2..5} (4 alike) : ManualSwitch  CurrentSetting=0
  Motor2Drone : MATLAB Function  TreatAsAtomicUnit=on
  MotorThrustCmd : MATLAB Function  TreatAsAtomicUnit=on
  Propellers : Subsystem
  Saturation{,1..3} (4 alike) : Saturate  UpperLimit=MaxThrust/4  LowerLimit=0
  Scope3 : Scope  NumInputPorts=2
  Scope7 : Scope  NumInputPorts=2
  Thrust : Outport
  Tq_R : Outport  Port=2
  Tq_P : Outport  Port=3
  Tq_Y : Outport  Port=4
  wires:
  MotorThrustCmd/3(BR_Cmd) -> Saturation2/1
  Manual Switch3/1 -> Motor2Drone/2(FL)
  Motor2Drone/3(Tq_P) -> Tq_P/1
  Thrust_Cmd/1 -> MotorThrustCmd/1(Thrust_Cmd)
  Saturation2/1 -> Manual Switch4/1, Scope7/1, Propellers/3(ref_Thrust2)  "BR_Thrust_Cmd"
  Tq_R_Cmd/1 -> MotorThrustCmd/2(Tq_R_Cmd)
  Manual Switch4/1 -> Motor2Drone/3(BR)
  Tq_Y_Cmd/1 -> MotorThrustCmd/4(Tq_Y_Cmd)
  Propellers/1(Thrust) -> Scope3/2, Manual Switch2/2  "FR_Thrust"
  Manual Switch5/1 -> Motor2Drone/4(BL)
  Tq_P_Cmd/1 -> MotorThrustCmd/3(Tq_P_Cmd)
  MotorThrustCmd/1(FR_Cmd) -> Saturation/1
  Motor2Drone/1(Thrust) -> Thrust/1
  Manual Switch2/1 -> Motor2Drone/1(FR)
  Length of Drone Arm/1 -> MotorThrustCmd/5(l), Motor2Drone/5(l)
  Saturation/1 -> Manual Switch2/1, Scope3/1, Propellers/1(ref_Thrust)  "FR_Thrust_Cmd"
  MotorThrustCmd/4(BL_Cmd) -> Saturation3/1
  Constant3/1 -> Motor2Drone/6(k), MotorThrustCmd/6(k)
  MotorThrustCmd/2(FL_Cmd) -> Saturation1/1
  Propellers/2(Thrust1) -> Manual Switch3/2  "FL_Thrust"
  Saturation3/1 -> Manual Switch5/1, Propellers/4(ref_Thrust3)  "BL_Thrust_Cmd"
  Saturation1/1 -> Propellers/2(ref_Thrust1), Manual Switch3/1  "FL_Thrust_Cmd"
  Motor2Drone/2(Tq_R) -> Tq_R/1
  Propellers/3(Thrust2) -> Scope7/2, Manual Switch4/2  "BR_Thrust"
  Motor2Drone/4(Tq_Y) -> Tq_Y/1
  Propellers/4(Thrust3) -> Manual Switch5/2  "BL_Thrust"

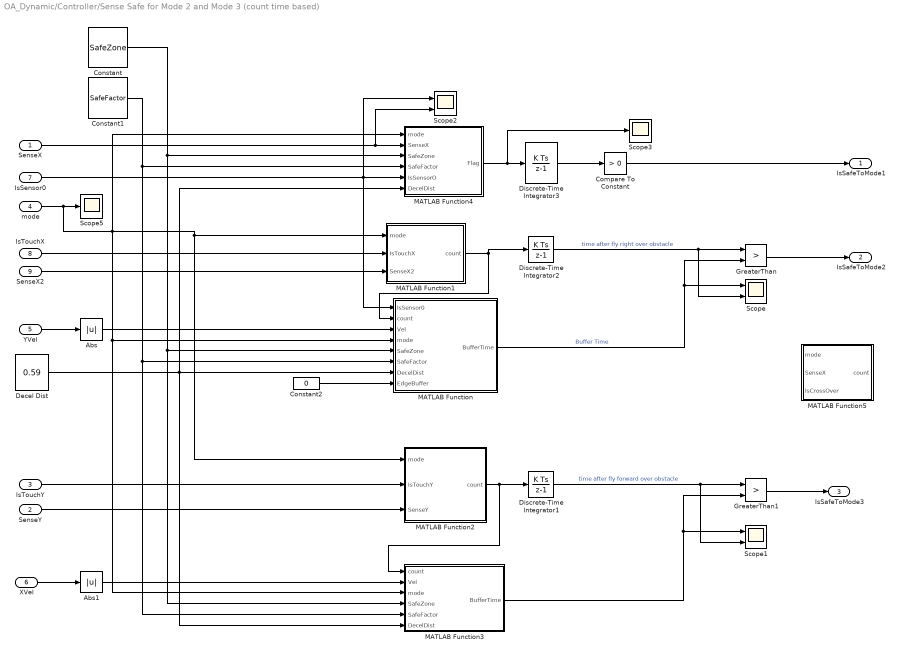
== system OA_Dynamic/Controller/Sense Safe for Mode 2 and Mode 3 (count time based) ==
  SenseX : Inport
  SenseY : Inport  Port=2
  IsTouchY : Inport  Port=3
  mode : Inport  Port=4
  YVel : Inport  Port=5
  XVel : Inport  Port=6
  IsSensor0 : Inport  Port=7
  IsTouchX : Inport  Port=8
  SenseX2 : Inport  Port=9
  Abs : Abs
  Abs1 : Abs
  Compare To Constant : simulink/Logic and Bit Operations/Compare To Constant  relop=>  const=0  OutDataTypeStr=boolean
  Constant : Constant  Value=SafeZone
  Constant1 : Constant  Value=SafeFactor
  Constant2 : Constant  Value=0
  Decel Dist : Constant  Value=0.59
  Discrete-Time Integrator1 : DiscreteIntegrator  SampleTime=ts  ICPrevOutput=DiscIntNeverNeededParam  ICPrevScaledInput=DiscIntNeverNeededParam
  Discrete-Time Integrator2 : DiscreteIntegrator  SampleTime=ts  ICPrevOutput=DiscIntNeverNeededParam  ICPrevScaledInput=DiscIntNeverNeededParam
  Discrete-Time Integrator3 : DiscreteIntegrator  SampleTime=ts  LimitOutput=on  UpperSaturationLimit=1  LowerSaturationLimit=0  ICPrevOutput=DiscIntNeverNeededParam  ICPrevScaledInput=DiscIntNeverNeededParam
  GreaterThan : RelationalOperator  Operator=>  OutDataTypeStr=boolean  RndMeth=Simplest
  GreaterThan1 : RelationalOperator  Operator=>  OutDataTypeStr=boolean  RndMeth=Simplest
  MATLAB Function : MATLAB Function  TreatAsAtomicUnit=on
  MATLAB Function1 : MATLAB Function  TreatAsAtomicUnit=on
  MATLAB Function2 : MATLAB Function  TreatAsAtomicUnit=on
  MATLAB Function3 : MATLAB Function  TreatAsAtomicUnit=on
  MATLAB Function4 : MATLAB Function  TreatAsAtomicUnit=on
  MATLAB Function5 : MATLAB Function  TreatAsAtomicUnit=on
  Scope : Scope  NumInputPorts=2
  Scope1 : Scope  NumInputPorts=2
  Scope2 : Scope  NumInputPorts=2
  Scope3 : Scope
  Scope5 : Scope
  IsSafeToMode1 : Outport
  IsSafeToMode2 : Outport  Port=2
  IsSafeToMode3 : Outport  Port=3
  wires:
  IsTouchY/1 -> MATLAB Function2/2(IsTouchY)
  SenseY/1 -> MATLAB Function2/3(SenseY)
  mode/1 -> MATLAB Function4/1(mode), MATLAB Function3/3(mode), MATLAB Function/4(mode), MATLAB Function2/1(mode), MATLAB Function1/1(mode), Scope5/1
  Discrete-Time Integrator2/1 -> GreaterThan/1, Scope/2  "time after fly right over obstacle"
  MATLAB Function1/1(count) -> Discrete-Time Integrator2/1, MATLAB Function/2(count)
  SenseX/1 -> MATLAB Function4/2(SenseX), Scope2/2
  Discrete-Time Integrator1/1 -> GreaterThan1/1, Scope1/2  "time after fly forward over obstacle"
  MATLAB Function2/1(count) -> MATLAB Function3/1(count), Discrete-Time Integrator1/1
  MATLAB Function/1(BufferTime) -> GreaterThan/2, Scope/1  "Buffer Time"
  YVel/1 -> Abs/1
  XVel/1 -> Abs1/1
  MATLAB Function3/1(BufferTime) -> GreaterThan1/2, Scope1/1
  Abs1/1 -> MATLAB Function3/2(Vel)
  MATLAB Function4/1(Flag) -> Scope3/1, Discrete-Time Integrator3/1
  Discrete-Time Integrator3/1 -> Compare To Constant/1
  Compare To Constant/1 -> IsSafeToMode1/1
  Constant/1 -> MATLAB Function3/4(SafeZone), MATLAB Function/5(SafeZone), MATLAB Function4/3(SafeZone)
  Constant1/1 -> MATLAB Function3/5(SafeFactor), MATLAB Function/6(SafeFactor), MATLAB Function4/4(SafeFactor)
  IsSensor0/1 -> Scope2/1, MATLAB Function/1(IsSensor0), MATLAB Function4/5(IsSensorO)
  Abs/1 -> MATLAB Function/3(Vel)
  GreaterThan1/1 -> IsSafeToMode3/1
  GreaterThan/1 -> IsSafeToMode2/1
  Decel Dist/1 -> MATLAB Function/7(DecelDist), MATLAB Function3/6(DecelDist), MATLAB Function4/6(DecelDist)
  Constant2/1 -> MATLAB Function/8(EdgeBuffer)
  IsTouchX/1 -> MATLAB Function1/2(IsTouchX)
  SenseX2/1 -> MATLAB Function1/3(SenseX2)

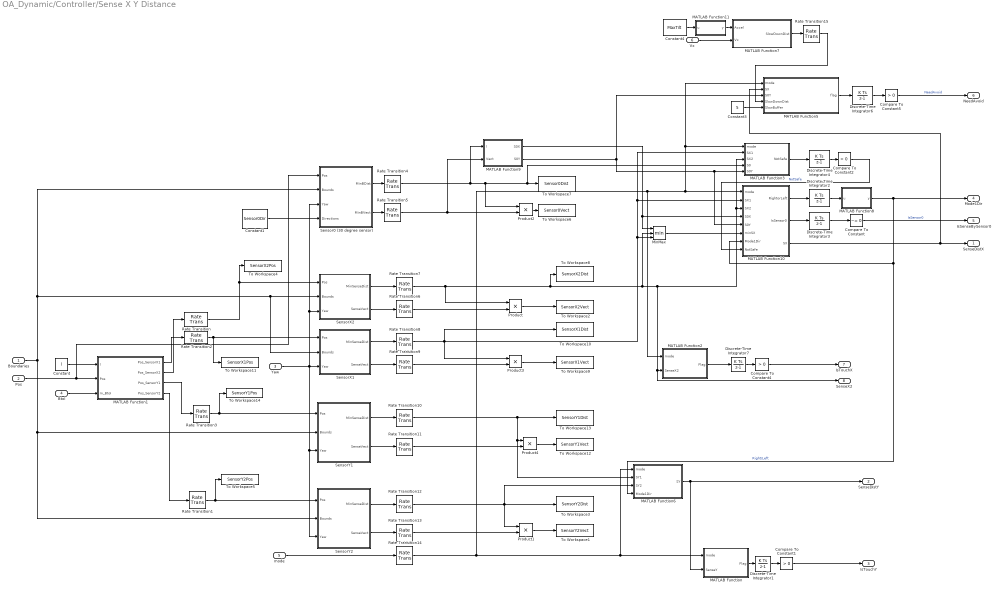
== system OA_Dynamic/Controller/Sense X Y Distance ==
  Boundaries : Inport
  Pos : Inport  Port=2
  Yaw : Inport  Port=3
  BtoI : Inport  Port=4
  mode : Inport  Port=5
  Vx : Inport  Port=6
  Compare To Constant : simulink/Logic and Bit Operations/Compare To Constant  relop=~=  const=0  OutDataTypeStr=boolean
  Compare To Constant{1..2,4..5} (4 alike) : simulink/Logic and Bit Operations/Compare To Constant  relop=>  const=0  OutDataTypeStr=boolean
  Constant : Constant  Value=l
  Constant1 : Constant  Value=Sensor0Dir
  Constant3 : Constant  Value=5
  Constant4 : Constant  Value=MaxTilt
  Discrete-Time Integrator1 : DiscreteIntegrator  SampleTime=0.1  ICPrevOutput=DiscIntNeverNeededParam  ICPrevScaledInput=DiscIntNeverNeededParam
  Discrete-Time Integrator2 : DiscreteIntegrator  SampleTime=0.1  LimitOutput=on  UpperSaturationLimit=1  LowerSaturationLimit=-1  ICPrevOutput=DiscIntNeverNeededParam  ICPrevScaledInput=DiscIntNeverNeededParam
  Discrete-Time Integrator3 : DiscreteIntegrator  SampleTime=0.1  LimitOutput=on  UpperSaturationLimit=1  LowerSaturationLimit=-1  ICPrevOutput=DiscIntNeverNeededParam  ICPrevScaledInput=DiscIntNeverNeededParam
  Discrete-Time Integrator4 : DiscreteIntegrator  SampleTime=0.1  LimitOutput=on  UpperSaturationLimit=1  LowerSaturationLimit=-1  ICPrevOutput=DiscIntNeverNeededParam  ICPrevScaledInput=DiscIntNeverNeededParam
  Discrete-Time Integrator6 : DiscreteIntegrator  SampleTime=0.1  LimitOutput=on  UpperSaturationLimit=1  LowerSaturationLimit=0  ICPrevOutput=DiscIntNeverNeededParam  ICPrevScaledInput=DiscIntNeverNeededParam
  Discrete-Time Integrator7 : DiscreteIntegrator  SampleTime=0.1  ICPrevOutput=DiscIntNeverNeededParam  ICPrevScaledInput=DiscIntNeverNeededParam
  MATLAB Function : MATLAB Function  TreatAsAtomicUnit=on
  MATLAB Function1 : MATLAB Function  TreatAsAtomicUnit=on
  MATLAB Function10 : MATLAB Function  TreatAsAtomicUnit=on
  MATLAB Function11 : MATLAB Function  TreatAsAtomicUnit=on
  MATLAB Function2 : MATLAB Function  TreatAsAtomicUnit=on
  MATLAB Function3 : MATLAB Function  TreatAsAtomicUnit=on
  MATLAB Function5 : MATLAB Function  TreatAsAtomicUnit=on
  MATLAB Function6 : MATLAB Function  TreatAsAtomicUnit=on
  MATLAB Function7 : MATLAB Function  TreatAsAtomicUnit=on
  MATLAB Function8 : MATLAB Function  TreatAsAtomicUnit=on
  MATLAB Function9 : MATLAB Function  TreatAsAtomicUnit=on
  MinMax : MinMax  Inputs=3
  Product{,1..4} (5 alike) : Product
  Rate Transition{,1..3} (4 alike) : RateTransition  OutPortSampleTime=ts
  Rate Transition{4..15} (12 alike) : RateTransition  OutPortSampleTime=0.1
  Sensor0 (30 degree sensor) : MATLAB Function  TreatAsAtomicUnit=on
  SensorX1 : MATLAB Function  TreatAsAtomicUnit=on
  SensorX2 : MATLAB Function  TreatAsAtomicUnit=on
  SensorY1 : MATLAB Function  TreatAsAtomicUnit=on
  SensorY2 : MATLAB Function  TreatAsAtomicUnit=on
  To Workspace1 : ToWorkspace  VariableName=SensorY2Vect  SampleTime=ts
  To Workspace10 : ToWorkspace  VariableName=SensorX1Dist  SampleTime=ts
  To Workspace11 : ToWorkspace  VariableName=SensorX1Pos  SampleTime=ts
  To Workspace12 : ToWorkspace  VariableName=SensorY1Vect  SampleTime=ts
  To Workspace13 : ToWorkspace  VariableName=SensorY1Dist  SampleTime=ts
  To Workspace14 : ToWorkspace  VariableName=SensorY1Pos  SampleTime=ts
  To Workspace2 : ToWorkspace  VariableName=SensorX2Vect  SampleTime=ts
  To Workspace3 : ToWorkspace  VariableName=SensorY2Dist  SampleTime=ts
  To Workspace4 : ToWorkspace  VariableName=SensorX2Pos  SampleTime=ts
  To Workspace5 : ToWorkspace  VariableName=SensorY2Pos  SampleTime=ts
  To Workspace6 : ToWorkspace  VariableName=Sensor0Vect  SampleTime=ts
  To Workspace7 : ToWorkspace  VariableName=Sensor0Dist  SampleTime=ts
  To Workspace8 : ToWorkspace  VariableName=SensorX2Dist  SampleTime=ts
  To Workspace9 : ToWorkspace  VariableName=SensorX1Vect  SampleTime=ts
  SenseDistX : Outport
  SenseDistY : Outport  Port=2
  IsTouchY : Outport  Port=3
  Mode1Dir : Outport  Port=4
  IsSenseBySensor0 : Outport  Port=5
  NeedAvoid : Outport  Port=6
  IsTouchX : Outport  Port=7
  SenseX2 : Outport  Port=8
  wires:
  mode/1 -> Rate Transition14/1
  Boundaries/1 -> Sensor0 (30 degree sensor)/2(Bounds), SensorX2/2(Bounds), SensorX1/2(Bounds), SensorY2/2(Bounds), SensorY1/2(Bounds)
  Yaw/1 -> SensorX1/3(Yaw), SensorY1/3(Yaw), SensorY2/3(Yaw), Sensor0 (30 degree sensor)/3(Yaw), SensorX2/3(Yaw)
  Pos/1 -> Sensor0 (30 degree sensor)/1(Pos), MATLAB Function1/2(Pos)
  Discrete-Time Integrator1/1 -> Compare To Constant1/1
  MATLAB Function/1(Flag) -> Discrete-Time Integrator1/1
  Compare To Constant1/1 -> IsTouchY/1
  Constant/1 -> MATLAB Function1/1(l)
  BtoI/1 -> MATLAB Function1/3(m_BtoI)
  MATLAB Function1/2(Pos_SensorX2) -> Rate Transition/1
  Product/1 -> To Workspace2/1
  SensorX2/2(SenseVect) -> Rate Transition6/1
  Product1/1 -> To Workspace1/1
  MATLAB Function1/4(Pos_SensorY2) -> Rate Transition1/1
  Rate Transition/1 -> To Workspace4/1, SensorX2/1(Pos)
  Rate Transition1/1 -> To Workspace5/1, SensorY2/1(Pos)
  Constant1/1 -> Sensor0 (30 degree sensor)/4(Directions)
  Sensor0 (30 degree sensor)/1(MinBDist) -> Rate Transition4/1
  Product2/1 -> To Workspace6/1
  Product3/1 -> To Workspace9/1
  MATLAB Function1/1(Pos_SensorX1) -> Rate Transition2/1
  Rate Transition2/1 -> To Workspace11/1, SensorX1/1(Pos)
  Rate Transition3/1 -> SensorY1/1(Pos), To Workspace14/1
  Product4/1 -> To Workspace12/1
  MATLAB Function1/3(Pos_SensorY1) -> Rate Transition3/1
  MATLAB Function6/1(SY) -> SenseDistY/1, MATLAB Function/2(SenseY)
  Discrete-Time Integrator2/1 -> MATLAB Function8/1(u)
  MATLAB Function8/1(y) -> MATLAB Function6/4(Mode1Dir), MATLAB Function10/7(Mode1Dir), Mode1Dir/1  "Right/Left"
  MATLAB Function9/2(S0Y) -> MATLAB Function5/3(S0Y), MATLAB Function3/5(S0Y), MATLAB Function10/5(S0Y)
  MATLAB Function10/1(RightorLeft) -> Discrete-Time Integrator2/1
  MATLAB Function10/2(IsSensor0) -> Discrete-Time Integrator3/1
  Discrete-Time Integrator3/1 -> Compare To Constant/1
  Compare To Constant/1 -> IsSenseBySensor0/1  "IsSensor0"
  MinMax/1 -> MATLAB Function10/6(minSX)
  MATLAB Function9/1(S0X) -> MinMax/1, MATLAB Function10/4(S0X)
  MATLAB Function3/1(NotSafe) -> Discrete-Time Integrator4/1
  Discrete-Time Integrator4/1 -> Compare To Constant2/1
  Compare To Constant2/1 -> MATLAB Function10/8(NotSafe)  "NotSafe"
  MATLAB Function10/3(SX) -> SenseDistX/1, MATLAB Function5/2(SX)
  Discrete-Time Integrator6/1 -> Compare To Constant5/1
  MATLAB Function5/1(flag) -> Discrete-Time Integrator6/1
  Compare To Constant5/1 -> NeedAvoid/1  "NeedAvoid"
  MATLAB Function7/1(SlowDownDist) -> Rate Transition15/1
  Vx/1 -> MATLAB Function7/2(Vx)
  Constant3/1 -> MATLAB Function5/5(SlowBuffer)
  Constant4/1 -> MATLAB Function11/1(u)
  MATLAB Function11/1(y) -> MATLAB Function7/1(Accel)
  Compare To Constant4/1 -> IsTouchX/1
  MATLAB Function2/1(Flag) -> Discrete-Time Integrator7/1
  Discrete-Time Integrator7/1 -> Compare To Constant4/1
  Rate Transition4/1 -> MATLAB Function3/4(S0), To Workspace7/1, Product2/1, MATLAB Function9/1(l)
  Sensor0 (30 degree sensor)/2(MinBVect) -> Rate Transition5/1
  Rate Transition5/1 -> MATLAB Function9/2(Vect), Product2/2
  Rate Transition6/1 -> Product/2
  SensorX2/1(MinSenseDist) -> Rate Transition7/1
  Rate Transition7/1 -> To Workspace8/1, SenseX2/1, MATLAB Function2/2(SenseX2), MATLAB Function10/3(SX2), MATLAB Function3/3(SX2), MinMax/2, Product/1
  SensorX1/1(MinSenseDist) -> Rate Transition8/1
  Rate Transition8/1 -> Product3/1, MinMax/3, MATLAB Function3/2(SX1), MATLAB Function10/2(SX1), To Workspace10/1
  SensorX1/2(SenseVect) -> Rate Transition9/1
  Rate Transition9/1 -> Product3/2
  Rate Transition10/1 -> MATLAB Function6/2(SY1), Product4/1, To Workspace13/1
  SensorY1/1(MinSenseDist) -> Rate Transition10/1
  SensorY1/2(SenseVect) -> Rate Transition11/1
  Rate Transition11/1 -> Product4/2
  Rate Transition12/1 -> MATLAB Function6/3(SY2), Product1/1, To Workspace3/1
  SensorY2/1(MinSenseDist) -> Rate Transition12/1
  SensorY2/2(SenseVect) -> Rate Transition13/1
  Rate Transition13/1 -> Product1/2
  Rate Transition14/1 -> MATLAB Function6/1(mode), MATLAB Function/1(mode), MATLAB Function5/1(mode), MATLAB Function3/1(mode), MATLAB Function10/1(mode), MATLAB Function2/1(mode)
  Rate Transition15/1 -> MATLAB Function5/4(SlowDownDist)

== system OA_Dynamic/Controller/Subsystem ==
  action : Inport
  Discrete-Time Integrator : DiscreteIntegrator  SampleTime=ts  ICPrevOutput=DiscIntNeverNeededParam  ICPrevScaledInput=DiscIntNeverNeededParam
  Gain : Gain  Gain=100
  Mode : Scope  NumInputPorts=2
  To Workspace7 : ToWorkspace  VariableName=Mode  SampleTime=ts
  mode : Outport
  wires:
  Discrete-Time Integrator/1 -> Gain/1
  Gain/1 -> Mode/2, To Workspace7/1, mode/1  "mode"
  action/1 -> Mode/1, Discrete-Time Integrator/1

== system OA_Dynamic/Controller/Subsystem1 ==
  mode : Inport
  Discrete-Time Integrator1 : DiscreteIntegrator  SampleTime=ts  ICPrevOutput=DiscIntNeverNeededParam  ICPrevScaledInput=DiscIntNeverNeededParam
  Discrete-Time Integrator2 : DiscreteIntegrator  SampleTime=ts  ICPrevOutput=DiscIntNeverNeededParam  ICPrevScaledInput=DiscIntNeverNeededParam
  GreaterThan : RelationalOperator  Operator=>  OutDataTypeStr=boolean  RndMeth=Simplest
  MATLAB Function1 : MATLAB Function  TreatAsAtomicUnit=on
  MATLAB Function2 : MATLAB Function  TreatAsAtomicUnit=on
  Scope : Scope
  Scope1 : Scope
  IsRecover : Outport
  wires:
  MATLAB Function1/1(y) -> Discrete-Time Integrator1/1
  GreaterThan/1 -> IsRecover/1
  mode/1 -> MATLAB Function2/1(u), MATLAB Function1/1(u)
  MATLAB Function2/1(y) -> Discrete-Time Integrator2/1
  Discrete-Time Integrator2/1 -> GreaterThan/1, Scope1/1  "time of mode 3"
  Discrete-Time Integrator1/1 -> GreaterThan/2, Scope/1  "time of mode 1"

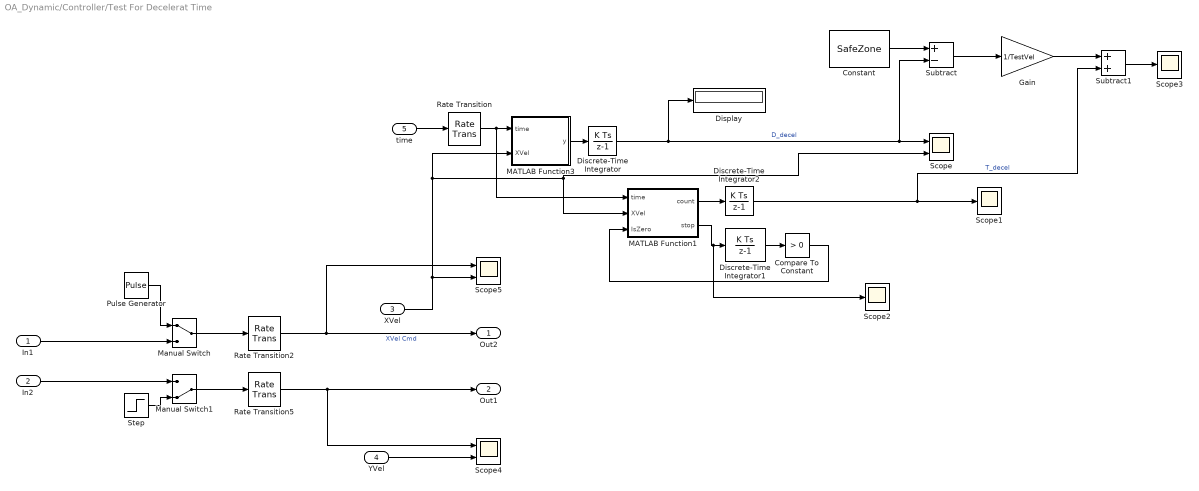
== system OA_Dynamic/Controller/Test For Decelerat Time ==
  In1 : Inport
  In2 : Inport  Port=2
  XVel : Inport  Port=3
  YVel : Inport  Port=4
  time : Inport  Port=5
  Compare To Constant : simulink/Logic and Bit Operations/Compare To Constant  relop=>  const=0  OutDataTypeStr=boolean
  Constant : Constant  Value=SafeZone
  Discrete-Time Integrator : DiscreteIntegrator  SampleTime=ts  ICPrevOutput=DiscIntNeverNeededParam  ICPrevScaledInput=DiscIntNeverNeededParam
  Discrete-Time Integrator1 : DiscreteIntegrator  SampleTime=ts  LimitOutput=on  UpperSaturationLimit=1  LowerSaturationLimit=0  ICPrevOutput=DiscIntNeverNeededParam  ICPrevScaledInput=DiscIntNeverNeededParam
  Discrete-Time Integrator2 : DiscreteIntegrator  SampleTime=ts  ICPrevOutput=DiscIntNeverNeededParam  ICPrevScaledInput=DiscIntNeverNeededParam
  Display : Display
  Gain : Gain  Gain=1/TestVel
  MATLAB Function1 : MATLAB Function  TreatAsAtomicUnit=on
  MATLAB Function3 : MATLAB Function  TreatAsAtomicUnit=on
  Manual Switch : ManualSwitch
  Manual Switch1 : ManualSwitch  CurrentSetting=0
  Pulse Generator : DiscretePulseGenerator  PulseType=Time based  Amplitude=TestVel  Period=40  PulseWidth=25  PhaseDelay=5
  Rate Transition : RateTransition  OutPortSampleTime=ts
  Rate Transition2 : RateTransition  OutPortSampleTime=ts
  Rate Transition5 : RateTransition  OutPortSampleTime=ts
  Scope : Scope  NumInputPorts=2
  Scope1 : Scope
  Scope2 : Scope
  Scope3 : Scope
  Scope4 : Scope  NumInputPorts=2
  Scope5 : Scope  NumInputPorts=2
  Step : Step  After=0  SampleTime=0
  Subtract : Sum  Inputs=+-
  Subtract1 : Sum
  Out2 : Outport
  Out1 : Outport  Port=2
  wires:
  In2/1 -> Manual Switch1/1
  Manual Switch/1 -> Rate Transition2/1
  Manual Switch1/1 -> Rate Transition5/1
  Rate Transition2/1 -> Out2/1, Scope5/1  "XVel Cmd"
  YVel/1 -> Scope4/2
  XVel/1 -> MATLAB Function3/2(XVel), MATLAB Function1/2(XVel), Scope/2, Scope5/2
  In1/1 -> Manual Switch/2
  Rate Transition5/1 -> Out1/1, Scope4/1
  time/1 -> Rate Transition/1
  MATLAB Function3/1(y) -> Discrete-Time Integrator/1
  Rate Transition/1 -> MATLAB Function1/1(time), MATLAB Function3/1(time)
  Discrete-Time Integrator/1 -> Display/1, Subtract/2, Scope/1  "D_decel"
  MATLAB Function1/1(count) -> Discrete-Time Integrator2/1
  MATLAB Function1/2(stop) -> Scope2/1, Discrete-Time Integrator1/1
  Discrete-Time Integrator1/1 -> Compare To Constant/1
  Compare To Constant/1 -> MATLAB Function1/3(IsZero)
  Discrete-Time Integrator2/1 -> Subtract1/2, Scope1/1  "T_decel"
  Pulse Generator/1 -> Manual Switch/1
  Step/1 -> Manual Switch1/2
  Constant/1 -> Subtract/1
  Subtract/1 -> Gain/1
  Gain/1 -> Subtract1/1
  Subtract1/1 -> Scope3/1

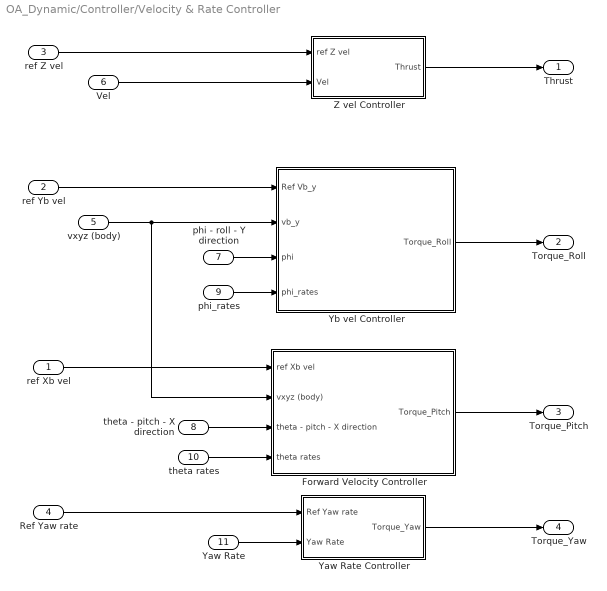
== system OA_Dynamic/Controller/Velocity & Rate Controller ==
  ref Xb vel : Inport
  ref Yb vel : Inport  Port=2
  ref Z vel : Inport  Port=3
  Ref Yaw rate : Inport  Port=4
  vxyz (body) : Inport  Port=5
  Vel : Inport  Port=6
  phi - roll - Y direction : Inport  Port=7
  theta - pitch - X direction : Inport  Port=8
  phi_rates : Inport  Port=9
  theta rates : Inport  Port=10
  Yaw Rate : Inport  Port=11
  Forward Velocity Controller : Subsystem
  Yaw Rate Controller : Subsystem
  Yb vel Controller : Subsystem
  Z vel Controller : Subsystem
  Thrust : Outport
  Torque_Roll : Outport  Port=2
  Torque_Pitch : Outport  Port=3
  Torque_Yaw : Outport  Port=4
  wires:
  Yb vel Controller/1(Torque_Roll) -> Torque_Roll/1
  Forward Velocity Controller/1(Torque_Pitch) -> Torque_Pitch/1
  theta - pitch - X direction/1 -> Forward Velocity Controller/3(theta - pitch - X direction)
  Z vel Controller/1(Thrust) -> Thrust/1
  phi - roll - Y direction/1 -> Yb vel Controller/3(phi)
  Ref Yaw rate/1 -> Yaw Rate Controller/1(Ref Yaw rate)
  ref Z vel/1 -> Z vel Controller/1(ref Z vel)
  vxyz (body)/1 -> Yb vel Controller/2(vb_y), Forward Velocity Controller/2(vxyz (body))
  Vel/1 -> Z vel Controller/2(Vel)
  theta rates/1 -> Forward Velocity Controller/4(theta rates)
  phi_rates/1 -> Yb vel Controller/4(phi_rates)
  Yaw Rate/1 -> Yaw Rate Controller/2(Yaw Rate)
  ref Xb vel/1 -> Forward Velocity Controller/1(ref Xb vel)
  Yaw Rate Controller/1(Torque_Yaw) -> Torque_Yaw/1
  ref Yb vel/1 -> Yb vel Controller/1(Ref Vb_y)

== system OA_Dynamic/Force and Environment1/Floor Contact Force ==
  Thrust : Inport
  m : Inport  Port=2
  Compare To Constant : simulink/Logic and Bit Operations/Compare To Constant  relop=>  const=0  OutDataTypeStr=boolean
  Discrete-Time Integrator : DiscreteIntegrator  SampleTime=-1  LimitOutput=on  UpperSaturationLimit=1  ICPrevOutput=DiscIntNeverNeededParam  ICPrevScaledInput=DiscIntNeverNeededParam
  MATLAB Function : MATLAB Function  TreatAsAtomicUnit=on
  MATLAB Function1 : MATLAB Function  TreatAsAtomicUnit=on
  Rate Transition : RateTransition  OutPortSampleTime=ts
  Scope : Scope
  Floor Contact Force : Outport
  wires:
  Rate Transition/1 -> MATLAB Function/1(Thrust)
  Discrete-Time Integrator/1 -> Compare To Constant/1
  MATLAB Function/1(DetectTakeOff) -> Discrete-Time Integrator/1
  Compare To Constant/1 -> MATLAB Function1/1(IsTakeOff), Scope/1
  Thrust/1 -> MATLAB Function1/2(Thrust), Rate Transition/1
  m/1 -> MATLAB Function/2(m), MATLAB Function1/3(m)
  MATLAB Function1/1(N) -> Floor Contact Force/1
